simulink model "six_plus_six_AcmsteeringV10_main"  (R2014a)
settings: Solver=FixedStepDiscrete  StartTime=0.0  StopTime=10.0  FixedStep=0.0005  RelTol=1e-3
InitFcn:
  | Veh_Par_wxt
values from neighbouring files (symbols this model uses):
  acc_spdctl = [0 100]    [Veh_Par_wxt.m]
  ag_thr = ecucoder_cal(ag_thr)    [Veh_Par_wxt.m]
  B = 1.8    [Veh_Par_wxt.m]
  bra_em = 100    [Veh_Par_wxt.m]
  bra_pre_gz2 = 100/3    (= 33.3333333333)    [Veh_Par_wxt.m]
  bra_pre_gz34 = 10/3    (= 3.33333333333)    [Veh_Par_wxt.m]
  bra_pre_yd = 10/2    (= 5)    [Veh_Par_wxt.m]
  brakepre_dem_data = [0 1 2 3 4 5 6 7 8 9 10]    [Veh_Par_wxt.m]
  brakeTrq_dem_data = [0 125 251 376 502 627 753 878 1004 1129 1255]    [Veh_Par_wxt.m]
  bratrq_max = 4*1255    (= 5020)    [Veh_Par_wxt.m]
  eff_tran = 0.9    [Veh_Par_wxt.m]
  ESP_switch = ecucoder_cal(ESP_switch)    [Veh_Par_wxt.m]
  G = Mass*g    (= 15696)    [Veh_Par_wxt.m]
  kd1 = ecucoder_cal(kd1)    [Veh_Par_wxt.m]
  kd2 = 0    [Veh_Par_wxt.m]
  ki1 = ecucoder_cal(ki1)    [Veh_Par_wxt.m]
  ki2 = 1    [Veh_Par_wxt.m]
  kp1 = ecucoder_cal(kp1)    [Veh_Par_wxt.m]
  kp2 = 300    [Veh_Par_wxt.m]
  L = L1+L2    (= 2.9)    [Veh_Par_wxt.m]
  premax = 100    [Veh_Par_wxt.m]
  Radius = 0.4572/2    (= 0.2286)    [Veh_Par_wxt.m]
  RC_switch = ecucoder_cal(RC_switch)    [Veh_Par_wxt.m]
  s_opt_yi = 0.15    [Veh_Par_wxt.m]
  s_opt_zhuan = 0.8    [Veh_Par_wxt.m]
  s_opt_zhuan_add = 0.05    [Veh_Par_wxt.m]
  s_opt_zhuan_table = [0.8 0.8 0.3 0.3]    [Veh_Par_wxt.m]
  spd_map_mot = [0 499.85 999.79 1500 2000 2500 3000 3500 4000 4500 4999.8 5999.8]    [Veh_Par_wxt.m]
  spd_spdctl = [0 500]    [Veh_Par_wxt.m]
  speed_thr_park = 5/3.6/Radius*tras_ratio*30/pi    (= 464.143899364)    [Veh_Par_wxt.m]
  TCS_switch = ecucoder_cal(TCS_switch)    [Veh_Par_wxt.m]
  tras_ratio = 8    [Veh_Par_wxt.m]
  trq_map_mot = [70.5 70.012 71.154 65.797 53.917 45.159 38.073 32.685 27.48 17.133 14.949 10.07]    [Veh_Par_wxt.m]
  trqmax_yd = 70.5    [Veh_Par_wxt.m]
  trqmax_zx = 70.5    [Veh_Par_wxt.m]
  trqmaxneg = -70.5    [Veh_Par_wxt.m]
  v_gain = 0.9    [Veh_Par_wxt.m]
  v_table = [0 5 20 100]    [Veh_Par_wxt.m]
  v_thr_park = 5    [Veh_Par_wxt.m]
  zhidong_bianmazhi = [-140000 750000]    [Veh_Par_wxt.m]
  zhidong_down = -140000    [Veh_Par_wxt.m]
  zhidong_up = 750000    [Veh_Par_wxt.m]
  zhidong_youmen = [0 100]    [Veh_Par_wxt.m]
  zhuanxiang_bianmazhi = [-400000 0 400000]    [Veh_Par_wxt.m]
  zhuanxiang_down = -400000    [Veh_Par_wxt.m]
  zhuanxiang_up = 400000    [Veh_Par_wxt.m]
  zhuanxiang_youmen = [-100 0 100]    [Veh_Par_wxt.m]
undefined symbols (not defined in the file or in its folder): ecucoder_acal, guzhang_lf, guzhang_lm, guzhang_lr, guzhang_rf, guzhang_rm, guzhang_rr, myFIS
libraries: simulink x979, ec5744lib x59, fuzblock x2
(part 24 of 27)

== system six_plus_six_AcmsteeringV10_main/MainControl/mode_control/forward/forward/Drive/Subsystem4 ==
  MCU2_3 : Inport
  Bus Selector : BusSelector  OutputSignals=MCU2_3MotorStallingFault,MCU2_3UdcDetectionFault,MCU2_3TempSensorFault,MCU2_3ActiveDischargingFault,MCU2_3ldcSensorFault,MCU2_3luSensorFault,MCU2_3lvSensorFault,MCU2_3FaultLevel,MCU2_3Controllerload,MCU2_3CanCommunicationFault,MCU2_3MemoryFault,MCU2_3DownratingFault,MCU2_3IGBTFault,MCU2_3MotorOverTemp,MCU2_3ControllerOverTemp,MCU2_3MotorOverSpeed,MCU2_3RotaryInverterFault,MCU2_3UnderVoltage,MCU2_3OverVoltage,MCU2_3MotorOverLoad
  Compare To Constant{,1..19} (20 alike) : simulink/Logic and Bit Operations/Compare To Constant  relop===  const=1  OutDataTypeStr=boolean
  Logical Operator : Logic  Operator=OR  Inputs=20  AllPortsSameDT=off  OutDataTypeStr=boolean
  guzhang_rm : Outport
  wires:
  MCU2_3/1 -> Bus Selector/1
  Bus Selector/1 -> Compare To Constant/1  "<MCU2_3MotorStallingFault>"
  Bus Selector/2 -> Compare To Constant1/1  "<MCU2_3UdcDetectionFault>"
  Bus Selector/3 -> Compare To Constant2/1  "<MCU2_3TempSensorFault>"
  Bus Selector/4 -> Compare To Constant3/1  "<MCU2_3ActiveDischargingFault>"
  Bus Selector/5 -> Compare To Constant4/1  "<MCU2_3ldcSensorFault>"
  Bus Selector/6 -> Compare To Constant5/1  "<MCU2_3luSensorFault>"
  Bus Selector/7 -> Compare To Constant6/1  "<MCU2_3lvSensorFault>"
  Bus Selector/8 -> Compare To Constant7/1  "<MCU2_3FaultLevel>"
  Bus Selector/13 -> Compare To Constant12/1  "<MCU2_3IGBTFault>"
  Bus Selector/14 -> Compare To Constant13/1  "<MCU2_3MotorOverTemp>"
  Bus Selector/10 -> Compare To Constant9/1  "<MCU2_3CanCommunicationFault>"
  Bus Selector/16 -> Compare To Constant15/1  "<MCU2_3MotorOverSpeed>"
  Bus Selector/11 -> Compare To Constant10/1  "<MCU2_3MemoryFault>"
  Bus Selector/15 -> Compare To Constant14/1  "<MCU2_3ControllerOverTemp>"
  Bus Selector/12 -> Compare To Constant11/1  "<MCU2_3DownratingFault>"
  Bus Selector/9 -> Compare To Constant8/1  "<MCU2_3Controllerload>"
  Bus Selector/18 -> Compare To Constant17/1  "<MCU2_3UnderVoltage>"
  Bus Selector/20 -> Compare To Constant19/1  "<MCU2_3MotorOverLoad>"
  Bus Selector/19 -> Compare To Constant18/1  "<MCU2_3OverVoltage>"
  Bus Selector/17 -> Compare To Constant16/1  "<MCU2_3RotaryInverterFault>"
  Compare To Constant9/1 -> Logical Operator/10
  Compare To Constant12/1 -> Logical Operator/13
  Compare To Constant11/1 -> Logical Operator/12
  Compare To Constant15/1 -> Logical Operator/16
  Compare To Constant8/1 -> Logical Operator/9
  Compare To Constant10/1 -> Logical Operator/11
  Compare To Constant13/1 -> Logical Operator/14
  Compare To Constant14/1 -> Logical Operator/15
  Compare To Constant1/1 -> Logical Operator/2
  Compare To Constant17/1 -> Logical Operator/18
  Compare To Constant16/1 -> Logical Operator/17
  Compare To Constant18/1 -> Logical Operator/19
  Compare To Constant19/1 -> Logical Operator/20
  Compare To Constant3/1 -> Logical Operator/4
  Compare To Constant2/1 -> Logical Operator/3
  Compare To Constant6/1 -> Logical Operator/7
  Compare To Constant4/1 -> Logical Operator/5
  Compare To Constant5/1 -> Logical Operator/6
  Compare To Constant7/1 -> Logical Operator/8
  Compare To Constant/1 -> Logical Operator/1
  Logical Operator/1 -> guzhang_rm/1

== system six_plus_six_AcmsteeringV10_main/MainControl/mode_control/forward/forward/Drive/Subsystem5 ==
  MCU2_5 : Inport
  Bus Selector : BusSelector  OutputSignals=MCU2_5MotorStallingFault,MCU2_5UdcDetectionFault,MCU2_5TempSensorFault,MCU2_5ActiveDischargingFault,MCU2_5ldcSensorFault,MCU2_5luSensorFault,MCU2_5lvSensorFault,MCU2_5FaultLevel,MCU2_5Controllerload,MCU2_5CanCommunicationFault,MCU2_5MemoryFault,MCU2_5DownratingFault,MCU2_5IGBTFault,MCU2_5MotorOverTemp,MCU2_5ControllerOverTemp,MCU2_5MotorOverSpeed,MCU2_5RotaryInverterFault,MCU2_5UnderVoltage,MCU2_5OverVoltage,MCU2_5MotorOverLoad
  Compare To Constant{,1..19} (20 alike) : simulink/Logic and Bit Operations/Compare To Constant  relop===  const=1  OutDataTypeStr=boolean
  Logical Operator : Logic  Operator=OR  Inputs=20  AllPortsSameDT=off  OutDataTypeStr=boolean
  guzhang_rr : Outport
  wires:
  Logical Operator/1 -> guzhang_rr/1
  Compare To Constant/1 -> Logical Operator/1
  Compare To Constant7/1 -> Logical Operator/8
  Compare To Constant5/1 -> Logical Operator/6
  Compare To Constant4/1 -> Logical Operator/5
  Compare To Constant6/1 -> Logical Operator/7
  Compare To Constant2/1 -> Logical Operator/3
  Compare To Constant3/1 -> Logical Operator/4
  Compare To Constant19/1 -> Logical Operator/20
  Compare To Constant18/1 -> Logical Operator/19
  Compare To Constant16/1 -> Logical Operator/17
  Compare To Constant17/1 -> Logical Operator/18
  Compare To Constant1/1 -> Logical Operator/2
  Compare To Constant14/1 -> Logical Operator/15
  Compare To Constant13/1 -> Logical Operator/14
  Compare To Constant10/1 -> Logical Operator/11
  Compare To Constant8/1 -> Logical Operator/9
  Compare To Constant15/1 -> Logical Operator/16
  Compare To Constant11/1 -> Logical Operator/12
  Compare To Constant12/1 -> Logical Operator/13
  Compare To Constant9/1 -> Logical Operator/10
  Bus Selector/17 -> Compare To Constant16/1  "<MCU2_5RotaryInverterFault>"
  Bus Selector/19 -> Compare To Constant18/1  "<MCU2_5OverVoltage>"
  Bus Selector/20 -> Compare To Constant19/1  "<MCU2_5MotorOverLoad>"
  Bus Selector/18 -> Compare To Constant17/1  "<MCU2_5UnderVoltage>"
  Bus Selector/9 -> Compare To Constant8/1  "<MCU2_5Controllerload>"
  Bus Selector/12 -> Compare To Constant11/1  "<MCU2_5DownratingFault>"
  Bus Selector/15 -> Compare To Constant14/1  "<MCU2_5ControllerOverTemp>"
  Bus Selector/11 -> Compare To Constant10/1  "<MCU2_5MemoryFault>"
  Bus Selector/16 -> Compare To Constant15/1  "<MCU2_5MotorOverSpeed>"
  Bus Selector/10 -> Compare To Constant9/1  "<MCU2_5CanCommunicationFault>"
  Bus Selector/14 -> Compare To Constant13/1  "<MCU2_5MotorOverTemp>"
  Bus Selector/13 -> Compare To Constant12/1  "<MCU2_5IGBTFault>"
  Bus Selector/8 -> Compare To Constant7/1  "<MCU2_5FaultLevel>"
  Bus Selector/7 -> Compare To Constant6/1  "<MCU2_5lvSensorFault>"
  Bus Selector/6 -> Compare To Constant5/1  "<MCU2_5luSensorFault>"
  Bus Selector/5 -> Compare To Constant4/1  "<MCU2_5ldcSensorFault>"
  Bus Selector/4 -> Compare To Constant3/1  "<MCU2_5ActiveDischargingFault>"
  Bus Selector/3 -> Compare To Constant2/1  "<MCU2_5TempSensorFault>"
  Bus Selector/2 -> Compare To Constant1/1  "<MCU2_5UdcDetectionFault>"
  Bus Selector/1 -> Compare To Constant/1  "<MCU2_5MotorStallingFault>"
  MCU2_5/1 -> Bus Selector/1

== matlab function six_plus_six_AcmsteeringV10_main/MainControl/mode_control/forward/forward/Drive/驱动防滑控制TCS/直行TCS/直行/HeartBeat4 ==
  data: life_pre input; life output
function life = fcn(life_pre)
%#codegen
life=single(life_pre+1);
if life>255
    life=single(0);
end
end

== matlab function six_plus_six_AcmsteeringV10_main/MainControl/mode_control/forward/forward/Drive/驱动防滑控制TCS/直行TCS/直行/HeartBeat5 ==
  data: life_pre input; life output
function life = fcn(life_pre)
%#codegen
life=single(life_pre+1);
if life>255
    life=single(0);
end
end

== matlab function six_plus_six_AcmsteeringV10_main/MainControl/mode_control/forward/forward/Brake/HeartBeat4 ==
  data: life_pre input; life output
function life = fcn(life_pre)
%#codegen
life=single(life_pre+1);
if life>255
    life=single(0);
end
end

== matlab function six_plus_six_AcmsteeringV10_main/MainControl/mode_control/neutral/neutral/HeartBeat ==
  data: life_pre input; life output
function life = fcn(life_pre)
%#codegen
life=single(life_pre+1);
if life>255
    life=single(0);
end
end

== matlab function six_plus_six_AcmsteeringV10_main/MainControl/mode_control/backward/backward/Brake/HeartBeat ==
  data: life_pre input; life output
function life = fcn(life_pre)
%#codegen
life=single(life_pre+1);
if life>255
    life=single(0);
end
end

== matlab function six_plus_six_AcmsteeringV10_main/MainControl/mode_control/backward/backward/Brake/Switch Case Action Subsystem/MATLAB Function5 ==
  data: bratrq_dem_lf input; bratrq_dem_lm input; bratrq_dem_lr input; bratrq_dem_rf input; bratrq_dem_rm input; bratrq_dem_rr input; pwr_chg_bat input; bratrq_mot_lf output; bratrq_mot_lm output; pwr_chg_bat1 input; pwr_chg_bat2 input; trqlimL_dig_lf input; bratrq_mot_lr output; bratrq_mot_rf output; bratrq_mot_rm output; bratrq_mot_rr output; trqlimL_dig_lm input; trqlimL_dig_lr input; trqlimL_dig_rf input; trqlimL_dig_rm input; trqlimL_dig_rr input; speed_act_lf input; speed_act_lm input; speed_act_lr input; speed_act_rf input; speed_act_rm input; speed_act_rr input; trqlim_map_lf input; brapre_out_l output; brapre_out_r output; trqlim_map_lm input; trqlim_map_lr input; trqlim_map_rf input; trqlim_map_rm input; trqlim_map_rr input; tras_ratio input; guzhang_lf input; guzhang_lm input; guzhang_lr input; guzhang_rf input; guzhang_rm input; guzhang_rr input
function [bratrq_mot_lf,bratrq_mot_lm,bratrq_mot_lr,bratrq_mot_rf,bratrq_mot_rm,bratrq_mot_rr,brapre_out_l,brapre_out_r] = fcn(bratrq_dem_lf,bratrq_dem_lm,bratrq_dem_lr,bratrq_dem_rf,bratrq_dem_rm,bratrq_dem_rr,pwr_chg_bat,pwr_chg_bat1,pwr_chg_bat2,trqlimL_dig_lf,trqlimL_dig_lm,trqlimL_dig_lr,trqlimL_dig_rf,trqlimL_dig_rm,trqlimL_dig_rr,speed_act_lf,speed_act_lm,speed_act_lr,speed_act_rf,speed_act_rm,speed_act_rr,trqlim_map_lf,trqlim_map_lm,trqlim_map_lr,trqlim_map_rf,trqlim_map_rm,trqlim_map_rr,tras_ratio,guzhang_lf,guzhang_lm,guzhang_lr,guzhang_rf,guzhang_rm,guzhang_rr)
%#codegen pid模块在外面做，里面进行十六种情况的判断，先看一下效果，不能再修改。前轴单独控制，后轴低选控制

bratrq_mot_lf1=single(bratrq_dem_lf/tras_ratio);
bratrq_mot_lf2=single(9549*(pwr_chg_bat/2)/speed_act_lf);
bratrq_mot_lf=single(min(trqlimL_dig_lf,min(bratrq_mot_lf1,bratrq_mot_lf2)));

bratrq_mot_lm1=single(bratrq_dem_lm/tras_ratio);
bratrq_mot_lm2=single(9549*(pwr_chg_bat1/2)/speed_act_lm);
bratrq_mot_lm=single(min(trqlimL_dig_lm,min(bratrq_mot_lm1,bratrq_mot_lm2)));

bratrq_mot_lr1=single(bratrq_dem_lr/tras_ratio);
bratrq_mot_lr2=single(9549*(pwr_chg_bat2/2)/speed_act_lr);
bratrq_mot_lr=single(min(trqlimL_dig_lr,min(bratrq_mot_lr1,bratrq_mot_lr2)));
 
bratrq_mot_rf1=single(bratrq_dem_rf/tras_ratio);
bratrq_mot_rf2=single(9549*(pwr_chg_bat/2)/speed_act_rf);
bratrq_mot_rf=single(min(trqlimL_dig_rf,min(bratrq_mot_rf1,bratrq_mot_rf2)));

bratrq_mot_rm1=single(bratrq_dem_rm/tras_ratio);
bratrq_mot_rm2=single(9549*(pwr_chg_bat1/2)/speed_act_rm);
bratrq_mot_rm=single(min(trqlimL_dig_rm,min(bratrq_mot_rm1,bratrq_mot_rm2)));

bratrq_mot_rr1=single(bratrq_dem_rr/tras_ratio);
bratrq_mot_rr2=single(9549*(pwr_chg_bat2/2)/speed_act_rr);
bratrq_mot_rr=single(min(trqlimL_dig_rr,min(bratrq_mot_rr1,bratrq_mot_rr2)));

brapre_out_l=single(((bratrq_dem_lf+bratrq_dem_lm+bratrq_dem_lr)-(bratrq_mot_lf+bratrq_mot_lm+bratrq_mot_lr)*tras_ratio)/3/150);
brapre_out_r=single(((bratrq_dem_rf+bratrq_dem_rm+bratrq_dem_rr)-(bratrq_mot_rf+bratrq_mot_rm+bratrq_mot_rr)*tras_ratio)/3/150);







bratrq_mot_lf=single(min(bratrq_mot_lf,trqlim_map_lf));%限一下最大值在外特性内，最小值大于0
bratrq_mot_lf=single(max(bratrq_mot_lf,0));
bratrq_mot_lr=single(min(bratrq_mot_lr,trqlim_map_lr));
bratrq_mot_lr=single(max(bratrq_mot_lr,0));
bratrq_mot_rf=single(min(bratrq_mot_rf,trqlim_map_rf));
bratrq_mot_rf=single(max(bratrq_mot_rf,0));
bratrq_mot_rr=single(min(bratrq_mot_rr,trqlim_map_rr));
bratrq_mot_rr=single(max(bratrq_mot_rr,0));

% brapre_out_l=brapre_out_l;
% brapre_out_r=brapre_out_r;
brapre_out_l=single(brapre_out_l*150/125);%第二辆车的制动压力与制动力的关系调整一下。
brapre_out_r=single(brapre_out_r*150/125);

if guzhang_lf==1
    bratrq_mot_lf=single(0);
end
if guzhang_lm==1
    bratrq_mot_lm=single(0);
end
if guzhang_lr==1
    bratrq_mot_lr=single(0);
end
if guzhang_rf==1
    bratrq_mot_rf=single(0);
end
if guzhang_rm==1
    bratrq_mot_rm=single(0);
end
if guzhang_rr==1
    bratrq_mot_rr=single(0);
end

end

== system six_plus_six_AcmsteeringV10_main/MainControl/mode_control/forward/forward/Drive/容错控制 ==
  trq_dem_l : Inport
  trq_dem_r : Inport  Port=2
  trqlim_lf : Inport  Port=3
  trqlim_lm : Inport  Port=4
  trqlim_lr : Inport  Port=5
  trqlim_rf : Inport  Port=6
  trqlim_rm : Inport  Port=7
  trqlim_rr : Inport  Port=8
  guzhang_lf : Inport  Port=9
  guzhang_lm : Inport  Port=10
  guzhang_lr : Inport  Port=11
  guzhang_rf : Inport  Port=12
  guzhang_rm : Inport  Port=13
  guzhang_rr : Inport  Port=14
  Constant : Constant  Value=bra_pre_gz2  OutDataTypeStr=single  SampleTime=-1
  Constant1 : Constant  Value=bra_pre_gz34  OutDataTypeStr=single  SampleTime=-1
  Constant11 : Constant  Value=RC_switch  OutDataTypeStr=single  SampleTime=-1
  Data Type Conversion{,1..5} (6 alike) : DataTypeConversion
  ECCalVar : Constant  InitFcn=ecucoder_acal;  Value=guzhang_lf  OutDataTypeStr=Inherit: Inherit via back propagation  SampleTime=-1
  ECCalVar1 : Constant  InitFcn=ecucoder_acal;  Value=guzhang_lm  OutDataTypeStr=Inherit: Inherit via back propagation  SampleTime=-1
  ECCalVar2 : Constant  InitFcn=ecucoder_acal;  Value=guzhang_lr  OutDataTypeStr=Inherit: Inherit via back propagation  SampleTime=-1
  ECCalVar3 : Constant  InitFcn=ecucoder_acal;  Value=guzhang_rf  OutDataTypeStr=Inherit: Inherit via back propagation  SampleTime=-1
  ECCalVar4 : Constant  InitFcn=ecucoder_acal;  Value=guzhang_rm  OutDataTypeStr=Inherit: Inherit via back propagation  SampleTime=-1
  ECCalVar5 : Constant  InitFcn=ecucoder_acal;  Value=guzhang_rr  OutDataTypeStr=Inherit: Inherit via back propagation  SampleTime=-1
  MATLAB Function : MATLAB Function  TreatAsAtomicUnit=on
  MATLAB Function5 : MATLAB Function  TreatAsAtomicUnit=on
  Terminator : Terminator
  trq_dem_lf : Outport
  trq_dem_lm : Outport  Port=2
  trq_dem_lr : Outport  Port=3
  trq_dem_rf : Outport  Port=4
  trq_dem_rm : Outport  Port=5
  trq_dem_rr : Outport  Port=6
  bra_pre_l : Outport  Port=7
  bra_pre_r : Outport  Port=8
  wires:
  trq_dem_r/1 -> MATLAB Function/2(trq_dem_r)
  trqlim_lr/1 -> MATLAB Function/5(trqlim_lr)
  trq_dem_l/1 -> MATLAB Function/1(trq_dem_l)
  trqlim_rf/1 -> MATLAB Function/6(trqlim_rf)
  trqlim_rr/1 -> MATLAB Function/8(trqlim_rr)
  trqlim_lf/1 -> MATLAB Function/3(trqlim_lf)
  MATLAB Function/1(trq_dem_lf) -> trq_dem_lf/1
  MATLAB Function/3(trq_dem_lr) -> trq_dem_lr/1
  MATLAB Function/4(trq_dem_rf) -> trq_dem_rf/1
  MATLAB Function/6(trq_dem_rr) -> trq_dem_rr/1
  MATLAB Function/7(bra_pre_l) -> bra_pre_l/1
  MATLAB Function/8(bra_pre_r) -> bra_pre_r/1
  Constant/1 -> MATLAB Function/15(bra_pre_gz2)
  Constant1/1 -> MATLAB Function/16(bra_pre_gz34)
  MATLAB Function/9(mode) -> Terminator/1
  trqlim_lm/1 -> MATLAB Function/4(trqlim_lm)
  trqlim_rm/1 -> MATLAB Function/7(trqlim_rm)
  MATLAB Function/2(trq_dem_lm) -> trq_dem_lm/1
  MATLAB Function/5(trq_dem_rm) -> trq_dem_rm/1
  Constant11/1 -> MATLAB Function5/1(RC_switch)
  MATLAB Function5/1(guzhang_lf1) -> Data Type Conversion/1
  MATLAB Function5/2(guzhang_lm1) -> Data Type Conversion1/1
  MATLAB Function5/3(guzhang_lr1) -> Data Type Conversion2/1
  MATLAB Function5/4(guzhang_rf1) -> Data Type Conversion3/1
  MATLAB Function5/6(guzhang_rr1) -> Data Type Conversion5/1
  MATLAB Function5/5(guzhang_rm1) -> Data Type Conversion4/1
  ECCalVar/1 -> MATLAB Function5/2(guzhang_lf)
  ECCalVar1/1 -> MATLAB Function5/3(guzhang_lm)
  ECCalVar2/1 -> MATLAB Function5/4(guzhang_lr)
  ECCalVar3/1 -> MATLAB Function5/5(guzhang_rf)
  ECCalVar4/1 -> MATLAB Function5/6(guzhang_rm)
  ECCalVar5/1 -> MATLAB Function5/7(guzhang_rr)
  Data Type Conversion/1 -> MATLAB Function/9(guzhang_lf)  "guzhang_lf"
  Data Type Conversion1/1 -> MATLAB Function/10(guzhang_lm)  "guzhang_lm"
  Data Type Conversion2/1 -> MATLAB Function/11(guzhang_lr)  "guzhang_lr"
  Data Type Conversion3/1 -> MATLAB Function/12(guzhang_rf)  "guzhang_rf"
  Data Type Conversion4/1 -> MATLAB Function/13(guzhang_rm)  "guzhang_rm"
  Data Type Conversion5/1 -> MATLAB Function/14(guzhang_rr)  "guzhang_rr"

== system six_plus_six_AcmsteeringV10_main/MainControl/mode_control/forward/forward/Drive/左右侧电机分配及功率限制 ==
  Trq_line_dem : Inport
  delta_T_dem : Inport  Port=2
  pwr_dis_bat : Inport  Port=3
  pwr_dis_bat1 : Inport  Port=4
  pwr_dis_bat2 : Inport  Port=5
  speed_act_lf : Inport  Port=6
  speed_act_lm : Inport  Port=7
  speed_act_lr : Inport  Port=8
  speed_act_rf : Inport  Port=9
  speed_act_rm : Inport  Port=10
  speed_act_rr : Inport  Port=11
  TrqLimU_dig_lf : Inport  Port=12
  TrqLimU_dig_lm : Inport  Port=13
  TrqLimU_dig_lr : Inport  Port=14
  TrqLimU_dig_rf : Inport  Port=15
  TrqLimU_dig_rm : Inport  Port=16
  TrqLimU_dig_rr : Inport  Port=17
  Add : Sum
  Add1 : Sum  Inputs=++++++
  Add2 : Sum  Inputs=+++
  Add3 : Sum  Inputs=+++
  Add4 : Sum  Inputs=+++
  Constant : Constant  Value=9549  OutDataTypeStr=single  SampleTime=-1
  Divide : Product  Inputs=**/
  Gain : Gain  Gain=1/6
  Gain1 : Gain  Gain=1/2
  Gain4 : Gain  Gain=1/2
  MATLAB Function : MATLAB Function  TreatAsAtomicUnit=on
  MinMax{,1..8} (9 alike) : MinMax  Inputs=2
  Subtract : Sum  Inputs=+-
  mot_map{,1..5} (6 alike) : Lookup_n-D  NumberOfTableDimensions=1  BreakpointsForDimension1=spd_map_mot  Table=trq_map_mot  InternalRulePriority=Speed  RndMeth=Simplest  InputSameDT=on
  trq_dem_l : Outport
  trq_dem_r : Outport  Port=2
  trqlim_lf : Outport  Port=3
  trqlim_lm : Outport  Port=4
  trqlim_lr : Outport  Port=5
  trqlim_rf : Outport  Port=6
  trqlim_rm : Outport  Port=7
  trqlim_rr : Outport  Port=8
  wires:
  speed_act_rf/1 -> Add1/4, mot_map2/1
  speed_act_lm/1 -> Add1/2, mot_map4/1
  speed_act_rr/1 -> Add1/6, mot_map3/1
  speed_act_lf/1 -> mot_map/1, Add1/1
  Add1/1 -> Gain/1
  Constant/1 -> Divide/1
  Gain/1 -> Divide/3
  Divide/1 -> MinMax/1
  Trq_line_dem/1 -> MinMax/2
  MinMax/1 -> Gain1/1
  Gain1/1 -> Subtract/1, Add/1
  delta_T_dem/1 -> Gain4/1, [delta_T_dem]
  Subtract/1 -> MinMax1/2
  MinMax1/1 -> MATLAB Function/2(trq_dem_l1)
  Add/1 -> MinMax2/2
  MinMax2/1 -> MATLAB Function/4(trq_dem_r1)
  mot_map3/1 -> MinMax3/1
  TrqLimU_dig_rr/1 -> MinMax3/2
  mot_map2/1 -> MinMax4/1
  TrqLimU_dig_rf/1 -> MinMax4/2
  mot_map1/1 -> MinMax5/1
  TrqLimU_dig_lr/1 -> MinMax5/2
  mot_map/1 -> MinMax6/1
  TrqLimU_dig_lf/1 -> MinMax6/2
  MinMax6/1 -> trqlim_lf/1, Add3/1
  MinMax5/1 -> trqlim_lr/1, Add3/3
  MinMax4/1 -> Add2/1, trqlim_rf/1
  MinMax3/1 -> Add2/3, trqlim_rr/1
  Add3/1 -> [trqlim_l]
  [trqlim_l] -> MATLAB Function/1(trqlim_l), MinMax1/1
  Add2/1 -> [trqlim_r]
  [trqlim_r] -> MATLAB Function/3(trqlim_r), MinMax2/1
  [delta_T_dem] -> MATLAB Function/5(delta_T_dem)
  MATLAB Function/1(trq_dem_l) -> trq_dem_l/1
  MATLAB Function/2(trq_dem_r) -> trq_dem_r/1
  Gain4/1 -> Add/2, Subtract/2
  speed_act_lr/1 -> Add1/3, mot_map1/1
  mot_map4/1 -> MinMax7/1
  TrqLimU_dig_lm/1 -> MinMax7/2
  MinMax7/1 -> Add3/2, trqlim_lm/1
  speed_act_rm/1 -> Add1/5, mot_map5/1
  mot_map5/1 -> MinMax8/1
  TrqLimU_dig_rm/1 -> MinMax8/2
  MinMax8/1 -> trqlim_rm/1, Add2/2
  pwr_dis_bat2/1 -> Add4/3
  pwr_dis_bat/1 -> Add4/1
  pwr_dis_bat1/1 -> Add4/2
  Add4/1 -> Divide/2

== system six_plus_six_AcmsteeringV10_main/MainControl/mode_control/forward/forward/Drive/目标直驶力矩确定模块 ==
  acc_dem : Inport
  TrqLimU_dig_lf : Inport  Port=2
  TrqLimU_dig_lm : Inport  Port=3
  TrqLimU_dig_lr : Inport  Port=4
  TrqLimU_dig_rf : Inport  Port=5
  TrqLimU_dig_rm : Inport  Port=6
  TrqLimU_dig_rr : Inport  Port=7
  speed_act_lf : Inport  Port=8
  speed_act_lm : Inport  Port=9
  speed_act_lr : Inport  Port=10
  speed_act_rf : Inport  Port=11
  speed_act_rm : Inport  Port=12
  speed_act_rr : Inport  Port=13
  Add : Sum  Inputs=++++++
  Constant : Constant  Value=3.6  OutDataTypeStr=single  SampleTime=-1
  Constant1 : Constant  Value=Radius  OutDataTypeStr=single  SampleTime=-1
  Constant2 : Constant  Value=30/pi  OutDataTypeStr=single  SampleTime=-1
  Divide : Product  Inputs=*//*
  Gain : Gain  Gain=1/100
  Gain1 : Gain  Gain=tras_ratio
  Ground : Ground
  MinMax{,1..5} (6 alike) : MinMax  Inputs=2
  Product : Product
  Terminator : Terminator
  mot_map{,1..5} (6 alike) : Lookup_n-D  NumberOfTableDimensions=1  BreakpointsForDimension1=spd_map_mot  Table=trq_map_mot  InternalRulePriority=Speed  RndMeth=Simplest  InputSameDT=on
  Trq_line_dem : Outport
  wires:
  Constant1/1 -> Divide/3
  Constant/1 -> Divide/2
  Constant2/1 -> Divide/4
  Divide/1 -> Gain1/1
  TrqLimU_dig_lf/1 -> MinMax/2
  mot_map/1 -> MinMax/1
  TrqLimU_dig_lm/1 -> MinMax1/2
  TrqLimU_dig_rm/1 -> MinMax2/2
  TrqLimU_dig_rr/1 -> MinMax3/2
  Add/1 -> Product/2
  acc_dem/1 -> Gain/1
  Gain/1 -> Product/1
  Ground/1 -> Divide/1
  Gain1/1 -> Terminator/1
  speed_act_lf/1 -> mot_map/1
  speed_act_lm/1 -> mot_map1/1
  speed_act_rm/1 -> mot_map2/1
  speed_act_rr/1 -> mot_map3/1
  mot_map1/1 -> MinMax1/1
  mot_map2/1 -> MinMax2/1
  mot_map3/1 -> MinMax3/1
  Product/1 -> Trq_line_dem/1
  TrqLimU_dig_lr/1 -> MinMax4/2
  mot_map4/1 -> MinMax4/1
  TrqLimU_dig_rf/1 -> MinMax5/2
  speed_act_lr/1 -> mot_map4/1
  speed_act_rf/1 -> mot_map5/1
  mot_map5/1 -> MinMax5/1
  MinMax1/1 -> Add/2
  MinMax/1 -> Add/1
  MinMax4/1 -> Add/3
  MinMax5/1 -> Add/4
  MinMax2/1 -> Add/5
  MinMax3/1 -> Add/6

== system six_plus_six_AcmsteeringV10_main/MainControl/mode_control/forward/forward/Drive/目标转向力矩确定模块 ==
  note: 左转为正，右转为负
  TrqLimU_dig_lf : Inport
  TrqLimU_dig_lm : Inport  Port=2
  TrqLimU_dig_lr : Inport  Port=3
  TrqLimU_dig_rf : Inport  Port=4
  TrqLimU_dig_rm : Inport  Port=5
  TrqLimU_dig_rr : Inport  Port=6
  steer_dem : Inport  Port=7
  umax : Inport  Port=8
  f : Inport  Port=9
  speed_act_lf : Inport  Port=10
  speed_act_lm : Inport  Port=11
  speed_act_lr : Inport  Port=12
  speed_act_rf : Inport  Port=13
  speed_act_rm : Inport  Port=14
  speed_act_rr : Inport  Port=15
  Add : Sum  Inputs=+++
  Add1 : Sum  Inputs=+++
  Add2 : Sum  Inputs=++++++
  Constant : Constant  Value=3.6  OutDataTypeStr=single  SampleTime=-1
  Constant1 : Constant  Value=Radius  OutDataTypeStr=single  SampleTime=-1
  Constant2 : Constant  Value=30/pi  OutDataTypeStr=single  SampleTime=-1
  Constant3 : Constant  Value=G  OutDataTypeStr=single  SampleTime=-1
  Constant4 : Constant  Value=L  OutDataTypeStr=single  SampleTime=-1
  Constant5 : Constant  Value=B  OutDataTypeStr=single  SampleTime=-1
  Constant6 : Constant  Value=eff_tran  OutDataTypeStr=single  SampleTime=-1
  Constant7 : Constant  Value=Radius  OutDataTypeStr=single  SampleTime=-1
  Constant8 : Constant  Value=ag_thr  OutDataTypeStr=single  SampleTime=-1
  Constant9 : Constant  Value=Radius  OutDataTypeStr=single  SampleTime=-1
  Divide : Product  Inputs=*//*
  Gain : Gain  Gain=1/100
  Gain1 : Gain  Gain=tras_ratio
  Gain10 : Gain  Gain=3.6
  Gain2 : Gain  Gain=tras_ratio  OutDataTypeStr=single
  Gain3 : Gain  Gain=1/tras_ratio
  Gain4 : Gain  Gain=tras_ratio  OutDataTypeStr=single
  Gain6 : Gain  Gain=1/6
  Gain7 : Gain  Gain=1/tras_ratio
  Gain8 : Gain  Gain=pi/30
  Gain9 : Gain  Gain=Radius
  Ground : Ground
  MATLAB Function : MATLAB Function  TreatAsAtomicUnit=on
  MATLAB Function1 : MATLAB Function  TreatAsAtomicUnit=on
  MATLAB Function2 : MATLAB Function  TreatAsAtomicUnit=on
  MinMax{,1..3,5..6} (6 alike) : MinMax  Inputs=2
  MinMax4 : MinMax  Function=max  Inputs=2
  Product : Product
  Terminator : Terminator
  mot_map{,1..5} (6 alike) : Lookup_n-D  NumberOfTableDimensions=1  BreakpointsForDimension1=spd_map_mot  Table=trq_map_mot  InternalRulePriority=Speed  RndMeth=Simplest  InputSameDT=on
  delta_Tsteer_dem : Outport
  wires:
  Gain/1 -> Product/1
  Product/1 -> Gain3/1
  [steer_dem] -> Gain/1
  MinMax3/1 -> Add1/2
  MinMax/1 -> Add/1
  MinMax2/1 -> Add1/1
  MinMax1/1 -> Add/2
  TrqLimU_dig_rm/1 -> MinMax3/2
  TrqLimU_dig_rf/1 -> MinMax2/2
  TrqLimU_dig_lm/1 -> MinMax1/2
  mot_map/1 -> MinMax/1
  TrqLimU_dig_lf/1 -> MinMax/2
  Divide/1 -> Gain1/1
  Constant2/1 -> Divide/4
  Constant/1 -> Divide/2
  Constant1/1 -> Divide/3
  steer_dem/1 -> [steer_dem], MATLAB Function/1(steer_dem)
  Constant3/1 -> [G], MATLAB Function/2(G)
  Constant4/1 -> [L], MATLAB Function/3(L)
  Constant5/1 -> [B], MATLAB Function/5(B)
  umax/1 -> [umax], MATLAB Function/4(umax)
  Add/1 -> Gain2/1
  Add1/1 -> Gain4/1
  Constant6/1 -> MATLAB Function/8(eff_tran)
  Constant7/1 -> MATLAB Function/9(Radius)
  f/1 -> MATLAB Function/10(f)
  MATLAB Function/1(Rturn_min) -> MinMax4/1
  [v_act] -> MATLAB Function1/1(v_act)
  Constant8/1 -> MATLAB Function1/2(ag_thr)
  MATLAB Function1/1(Rturn_min_ag) -> MinMax4/2
  [umax] -> MATLAB Function2/1(umax)
  [G] -> MATLAB Function2/2(G)
  [L] -> MATLAB Function2/3(L)
  [B] -> MATLAB Function2/4(B)
  Constant9/1 -> MATLAB Function2/5(Radius)
  MinMax4/1 -> MATLAB Function2/6(Rturn_min_xy)
  MATLAB Function2/1(delta_Tsteer_max) -> Product/2
  Ground/1 -> Divide/1
  Gain2/1 -> MATLAB Function/6(Tpeak_L)
  Gain4/1 -> MATLAB Function/7(Tpeak_R)
  speed_act_lm/1 -> Add2/2, mot_map2/1
  speed_act_rf/1 -> Add2/4, mot_map3/1
  speed_act_rm/1 -> Add2/5, mot_map4/1
  Gain1/1 -> Terminator/1
  speed_act_lf/1 -> Add2/1, mot_map/1
  mot_map2/1 -> MinMax1/1
  mot_map3/1 -> MinMax2/1
  mot_map4/1 -> MinMax3/1
  Gain3/1 -> delta_Tsteer_dem/1
  MinMax5/1 -> Add/3
  TrqLimU_dig_lr/1 -> MinMax5/2
  speed_act_lr/1 -> Add2/3, mot_map1/1
  mot_map1/1 -> MinMax5/1
  MinMax6/1 -> Add1/3
  TrqLimU_dig_rr/1 -> MinMax6/2
  speed_act_rr/1 -> Add2/6, mot_map5/1
  mot_map5/1 -> MinMax6/1
  Add2/1 -> Gain6/1
  Gain6/1 -> Gain7/1
  Gain7/1 -> Gain8/1
  Gain8/1 -> Gain9/1
  Gain9/1 -> Gain10/1
  Gain10/1 -> [v_act]

== system six_plus_six_AcmsteeringV10_main/MainControl/mode_control/forward/forward/Drive/路面状况识别模块 ==
  In1 : Inport
  miu : Inport  Port=2
  slip_ratio : Inport  Port=3
  Signals : Inport  Port=4
  1-D Lookup Table : Lookup_n-D  NumberOfTableDimensions=1  BreakpointsForDimension1=v_table  Table=s_opt_zhuan_table  InternalRulePriority=Speed  RndMeth=Simplest  InputSameDT=on
  Abs{11..14,19..20} (6 alike) : Abs  OutDataTypeStr=single
  Bus Selector8 : BusSelector  OutputSignals=MOTOR.MOTOR1.MCU0.MCU0_SpeedFdk,MOTOR.MOTOR3.MCU0_2.MCU0_2SpeedFdk,MOTOR.MOTOR5.MCU0_4.MCU0_4SpeedFdk,MOTOR.MOTOR2.MCU0_1.MCU0_1SpeedFdk,MOTOR.MOTOR4.MCU0_3.MCU0_3SpeedFdk,MOTOR.MOTOR6.MCU0_5.MCU0_5SpeedFdk
  Constant : Constant  Value=0.9  OutDataTypeStr=single  SampleTime=-1
  Constant1 : Constant  Value=0.05  OutDataTypeStr=single  SampleTime=-1
  Constant2 : Constant  Value=s_opt_zhuan  OutDataTypeStr=single  SampleTime=-1
  Constant3 : Constant  Value=s_opt_yi  OutDataTypeStr=single  SampleTime=-1
  Gain1 : Gain  Gain=1/tras_ratio
  Gain2 : Gain  Gain=pi/30
  Gain3 : Gain  Gain=Radius
  Gain4 : Gain  Gain=3.6
  Gain5 : Gain  Gain=v_gain
  MinMax : MinMax  Inputs=6
  Terminator{,1..3} (4 alike) : Terminator
  路面识别模块 : Subsystem  Commented=on
  umax : Outport
  f : Outport  Port=2
  s_opt_zhuan : Outport  Port=3
  s_opt_yi : Outport  Port=4
  wires:
  Constant/1 -> umax/1
  Constant1/1 -> f/1
  Constant2/1 -> Terminator3/1
  Constant3/1 -> s_opt_yi/1
  In1/1 -> Terminator/1
  miu/1 -> 路面识别模块/1(miu)
  slip_ratio/1 -> 路面识别模块/2(slip_ratio)
  路面识别模块/1(best_slip_ratio) -> Terminator1/1
  路面识别模块/2(max_miu) -> Terminator2/1
  Signals/1 -> Bus Selector8/1
  Abs12/1 -> MinMax/2
  Abs11/1 -> MinMax/1
  Abs13/1 -> MinMax/3
  Abs14/1 -> MinMax/4
  Abs19/1 -> MinMax/5
  Abs20/1 -> MinMax/6
  Bus Selector8/2 -> Abs12/1  "<MCU0_2SpeedFdk>"
  Bus Selector8/1 -> Abs11/1  "<MCU0_SpeedFdk>"
  Bus Selector8/3 -> Abs13/1  "<MCU0_4SpeedFdk>"
  Bus Selector8/4 -> Abs14/1  "<MCU0_1SpeedFdk>"
  Bus Selector8/5 -> Abs19/1  "<MCU0_3SpeedFdk>"
  Bus Selector8/6 -> Abs20/1  "<MCU0_5SpeedFdk>"
  MinMax/1 -> Gain1/1
  Gain1/1 -> Gain2/1
  Gain2/1 -> Gain3/1
  Gain3/1 -> Gain4/1
  Gain4/1 -> Gain5/1
  Gain5/1 -> 1-D Lookup Table/1
  1-D Lookup Table/1 -> s_opt_zhuan/1

== system six_plus_six_AcmsteeringV10_main/MainControl/mode_control/forward/forward/Drive/车辆稳定性控制 ==
  note: 加速度向左为正
  acc_y : Inport
  Action Port : ActionPort  ActionType=case
  Abs : Abs
  Add10 : Sum  Inputs=+-+
  Add2 : Sum  Inputs=+++
  Constant : Constant  Value=ag_thr  OutDataTypeStr=single  SampleTime=-1
  Constant1 : Constant  OutDataTypeStr=int8  SampleTime=-1
  Constant2 : Constant  Value=-1  OutDataTypeStr=int8  SampleTime=-1
  Constant3 : Constant  Value=ESP_switch  OutDataTypeStr=single  SampleTime=-1
  Constant4 : Constant  Value=0  OutDataTypeStr=single  SampleTime=-1
  Gain20 : Gain  Gain=2
  Gain3 : Gain  Gain=1/tras_ratio
  Gain5 : Gain  Gain=kp1  OutDataTypeStr=single
  Gain6 : Gain  Gain=ki1  OutDataTypeStr=single
  Gain7 : Gain  Gain=kd1  OutDataTypeStr=single
  Memory{3..5,13} (4 alike) : Memory  InheritSampleTime=on
  Product : Product  OutDataTypeStr=single
  Subtract1 : Sum  Inputs=+-
  Subtract5 : Sum
  Sum : Sum  Inputs=|+-
  Switch : Switch
  Switch1 : Switch  Criteria=u2 > Threshold  Threshold=0.5
  delta_Twending_dem : Outport
  wires:
  Constant/1 -> Sum/1
  acc_y/1 -> Switch/2, Abs/1  "acc_y"
  Constant1/1 -> Switch/1
  Constant2/1 -> Switch/3
  Switch/1 -> Product/2
  Product/1 -> Gain3/1
  Constant3/1 -> Switch1/2
  Switch1/1 -> delta_Twending_dem/1  "delta_Twending_dem"
  Constant4/1 -> Switch1/3
  Sum/1 -> Memory4/1, Add10/1, Gain6/1, Memory3/1, Subtract1/1
  Gain5/1 -> Add2/1
  Gain6/1 -> Add2/2
  Memory3/1 -> Subtract1/2
  Add10/1 -> Gain7/1
  Gain20/1 -> Add10/2
  Memory5/1 -> Add10/3
  Gain7/1 -> Add2/3
  Subtract1/1 -> Gain5/1
  Memory4/1 -> Memory5/1, Gain20/1
  Add2/1 -> Subtract5/1
  Subtract5/1 -> Product/1, Memory13/1
  Memory13/1 -> Subtract5/2
  Abs/1 -> Sum/2
  Gain3/1 -> Switch1/1

== system six_plus_six_AcmsteeringV10_main/MainControl/mode_control/forward/forward/Drive/车辆稳定性控制1 ==
  Action Port : ActionPort  ActionType=case
  Constant4 : Constant  Value=0  OutDataTypeStr=single  SampleTime=-1
  1 : Outport
  wires:
  Constant4/1 -> 1/1

== system six_plus_six_AcmsteeringV10_main/MainControl/mode_control/forward/forward/Drive/驱动防滑控制TCS ==
  trq_dem_lf : Inport
  trq_dem_lm : Inport  Port=2
  trq_dem_lr : Inport  Port=3
  trq_dem_rf : Inport  Port=4
  trq_dem_rm : Inport  Port=5
  trq_dem_rr : Inport  Port=6
  bra_pre_l : Inport  Port=7
  bra_pre_r : Inport  Port=8
  speed_act_lf : Inport  Port=9
  speed_act_lm : Inport  Port=10
  speed_act_lr : Inport  Port=11
  speed_act_rf : Inport  Port=12
  speed_act_rm : Inport  Port=13
  speed_act_rr : Inport  Port=14
  v_act : Inport  Port=15
  brake_dem : Inport  Port=16
  s_opt_zhuan : Inport  Port=17
  Signals : Inport  Port=18
  直行TCS : Subsystem  TreatAsAtomicUnit=on
  forward_dem : Outport
  wires:
  直行TCS/1(forward_dem) -> forward_dem/1
  trq_dem_lf/1 -> 直行TCS/1(trq_dem_lf)
  trq_dem_lm/1 -> 直行TCS/2(trq_dem_lm)
  trq_dem_lr/1 -> 直行TCS/3(trq_dem_lr)
  trq_dem_rf/1 -> 直行TCS/4(trq_dem_rf)
  trq_dem_rm/1 -> 直行TCS/5(trq_dem_rm)
  trq_dem_rr/1 -> 直行TCS/6(trq_dem_rr)
  bra_pre_l/1 -> 直行TCS/7(bra_pre_l)
  bra_pre_r/1 -> 直行TCS/8(bra_pre_r)
  brake_dem/1 -> 直行TCS/16(brake_dem)
  Signals/1 -> 直行TCS/18(Signals)
  speed_act_rr/1 -> 直行TCS/14(speed_act_rr)
  speed_act_rm/1 -> 直行TCS/13(speed_act_rm)
  v_act/1 -> 直行TCS/15(v_act)
  speed_act_rf/1 -> 直行TCS/12(speed_act_rf)
  speed_act_lr/1 -> 直行TCS/11(speed_act_lr)
  speed_act_lm/1 -> 直行TCS/10(speed_act_lm)
  speed_act_lf/1 -> 直行TCS/9(speed_act_lf)
  s_opt_zhuan/1 -> 直行TCS/17(s_opt_zhuan)

== system six_plus_six_AcmsteeringV10_main/MainControl/mode_control/backward/backward/Drive/路面状况识别模块/路面识别模块 ==
  miu : Inport
  slip_ratio : Inport  Port=2
  Add : Sum  Inputs=+++++
  Add1 : Sum  Inputs=+++++
  Add2 : Sum  Inputs=+++++
  Demux : Demux  Outputs=5
  Display : Display
  Display1 : Display
  Display2 : Display
  Divide : Product  Inputs=*/
  Divide1 : Product  Inputs=/*
  Fuzzy Logic Controller : fuzblock/Fuzzy Logic  Controller  fis=[myFIS]
  Gain : Gain  Gain=0.03
  Gain1 : Gain  Gain=0.05
  Gain2 : Gain  Gain=0.06
  Gain3 : Gain  Gain=0.19
  Gain4 : Gain  Gain=0.14
  Gain5 : Gain  Gain=0.34
  Gain6 : Gain  Gain=0.13
  Gain7 : Gain  Gain=0.80
  Gain8 : Gain  Gain=0.17
  Gain9 : Gain  Gain=1.17
  Mux : Mux  Inputs=2
  Scope : Scope
  Scope1 : Scope
  Scope2 : Scope
      settings: SaveName=ScopeData2
  best_slip_ratio : Outport
  max_miu : Outport  Port=2
  wires:
  Gain6/1 -> Add/4
  Gain4/1 -> Add/3
  Gain/1 -> Add/1
  Demux/1 -> Add1/1, Gain1/1, Gain/1
  Demux/4 -> Add1/4, Gain6/1, Gain7/1
  Add1/1 -> Divide1/1, Divide/2, Display2/1, Scope/1
  Gain5/1 -> Add2/3
  Gain1/1 -> Add2/1
  Gain9/1 -> Add2/5
  Divide/1 -> Display/1, Scope1/1, best_slip_ratio/1
  Gain7/1 -> Add2/4
  Add/1 -> Divide/1
  Gain2/1 -> Add/2
  Gain8/1 -> Add/5
  Demux/2 -> Add1/2, Gain3/1, Gain2/1
  Mux/1 -> Fuzzy Logic Controller/1
  Fuzzy Logic Controller/1 -> Demux/1
  Demux/3 -> Add1/3, Gain5/1, Gain4/1
  Gain3/1 -> Add2/2
  Add2/1 -> Divide1/2
  Divide1/1 -> Display1/1, Scope2/1, max_miu/1
  Demux/5 -> Add1/5, Gain9/1, Gain8/1
  slip_ratio/1 -> Mux/1
  miu/1 -> Mux/2

== system six_plus_six_AcmsteeringV10_main/MainControl/mode_control/backward/backward/Drive/驱动防滑控制TCS/直行TCS ==
  trq_dem_lf : Inport
  trq_dem_lm : Inport  Port=2
  trq_dem_lr : Inport  Port=3
  trq_dem_rf : Inport  Port=4
  trq_dem_rm : Inport  Port=5
  trq_dem_rr : Inport  Port=6
  bra_pre_l : Inport  Port=7
  bra_pre_r : Inport  Port=8
  speed_act_lf : Inport  Port=9
  speed_act_lm : Inport  Port=10
  speed_act_lr : Inport  Port=11
  speed_act_rf : Inport  Port=12
  speed_act_rm : Inport  Port=13
  speed_act_rr : Inport  Port=14
  v_act : Inport  Port=15
  brake_dem : Inport  Port=16
  s_opt_zhuan : Inport  Port=17
  Signals : Inport  Port=18
  Saturation{,1..5} (6 alike) : Saturate  UpperLimit=2  LowerLimit=0  OutDataTypeStr=single
  Subsystem : Subsystem
  Subsystem1 : Subsystem
  Subsystem2 : Subsystem
  Subsystem3 : Subsystem
  Subsystem4 : Subsystem
  Subsystem5 : Subsystem
  Subsystem6 : Subsystem
  Subsystem7 : Subsystem
  直行 : Subsystem  TreatAsAtomicUnit=on
  backward_dem : Outport
  wires:
  直行/1(backward_dem) -> backward_dem/1
  bra_pre_r/1 -> 直行/8(bra_pre_r)
  bra_pre_l/1 -> 直行/7(bra_pre_l)
  trq_dem_rf/1 -> 直行/4(trq_dem_rf)
  trq_dem_lf/1 -> 直行/1(trq_dem_lf)
  trq_dem_lr/1 -> 直行/3(trq_dem_lr)
  trq_dem_lm/1 -> 直行/2(trq_dem_lm)
  trq_dem_rm/1 -> 直行/5(trq_dem_rm)
  trq_dem_rr/1 -> 直行/6(trq_dem_rr)
  brake_dem/1 -> 直行/15(brake_dem)
  Signals/1 -> 直行/17(Signals)
  Subsystem/1(s_act_lf) -> Saturation/1
  speed_act_lf/1 -> Subsystem6/1(speed_act_lf), Subsystem/1(speed_act_lf)
  Saturation/1 -> 直行/9(s_act_lf)
  Subsystem1/1(s_act_lm) -> Saturation1/1
  Saturation1/1 -> 直行/10(s_act_lm)
  speed_act_lm/1 -> Subsystem6/2(speed_act_lm), Subsystem1/1(speed_act_lm)
  Subsystem2/1(s_act_lr) -> Saturation2/1
  Saturation2/1 -> 直行/11(s_act_lr)
  speed_act_lr/1 -> Subsystem6/3(speed_act_lr), Subsystem2/1(speed_act_lr)
  Subsystem3/1(s_act_rf) -> Saturation3/1
  Saturation3/1 -> 直行/12(s_act_rf)
  speed_act_rf/1 -> Subsystem7/1(speed_act_rf), Subsystem3/1(speed_act_rf)
  Subsystem4/1(s_act_rm) -> Saturation4/1
  speed_act_rm/1 -> Subsystem7/2(speed_act_rm), Subsystem4/1(speed_act_rm)
  Saturation4/1 -> 直行/13(s_act_rm)
  Subsystem5/1(s_act_rr) -> Saturation5/1
  Saturation5/1 -> 直行/14(s_act_rr)
  speed_act_rr/1 -> Subsystem7/3(speed_act_rr), Subsystem5/1(speed_act_rr)
  s_opt_zhuan/1 -> 直行/16(s_opt_zhuan)
  Subsystem6/1(v_act_l) -> Subsystem1/2(v_act), Subsystem/2(v_act), Subsystem2/2(v_act)
  Subsystem7/1(v_act_r) -> Subsystem3/2(v_act), Subsystem4/2(v_act), Subsystem5/2(v_act)

== system six_plus_six_AcmsteeringV10_main/MainControl/mode_control/forward/forward/Drive/路面状况识别模块/路面识别模块 ==
  miu : Inport
  slip_ratio : Inport  Port=2
  Add : Sum  Inputs=+++++
  Add1 : Sum  Inputs=+++++
  Add2 : Sum  Inputs=+++++
  Demux : Demux  Outputs=5
  Display : Display
  Display1 : Display
  Display2 : Display
  Divide : Product  Inputs=*/
  Divide1 : Product  Inputs=/*
  Fuzzy Logic Controller : fuzblock/Fuzzy Logic  Controller  fis=[myFIS]
  Gain : Gain  Gain=0.03
  Gain1 : Gain  Gain=0.05
  Gain2 : Gain  Gain=0.06
  Gain3 : Gain  Gain=0.19
  Gain4 : Gain  Gain=0.14
  Gain5 : Gain  Gain=0.34
  Gain6 : Gain  Gain=0.13
  Gain7 : Gain  Gain=0.80
  Gain8 : Gain  Gain=0.17
  Gain9 : Gain  Gain=1.17
  Mux : Mux  Inputs=2
  Scope : Scope
  Scope1 : Scope
  Scope2 : Scope
      settings: SaveName=ScopeData2
  best_slip_ratio : Outport
  max_miu : Outport  Port=2
  wires:
  Gain6/1 -> Add/4
  Gain4/1 -> Add/3
  Gain/1 -> Add/1
  Demux/1 -> Add1/1, Gain1/1, Gain/1
  Demux/4 -> Add1/4, Gain6/1, Gain7/1
  Add1/1 -> Divide1/1, Divide/2, Display2/1, Scope/1
  Gain5/1 -> Add2/3
  Gain1/1 -> Add2/1
  Gain9/1 -> Add2/5
  Divide/1 -> Display/1, Scope1/1, best_slip_ratio/1
  Gain7/1 -> Add2/4
  Add/1 -> Divide/1
  Gain2/1 -> Add/2
  Gain8/1 -> Add/5
  Demux/2 -> Add1/2, Gain3/1, Gain2/1
  Mux/1 -> Fuzzy Logic Controller/1
  Fuzzy Logic Controller/1 -> Demux/1
  Demux/3 -> Add1/3, Gain5/1, Gain4/1
  Gain3/1 -> Add2/2
  Add2/1 -> Divide1/2
  Divide1/1 -> Display1/1, Scope2/1, max_miu/1
  Demux/5 -> Add1/5, Gain9/1, Gain8/1
  slip_ratio/1 -> Mux/1
  miu/1 -> Mux/2

== system six_plus_six_AcmsteeringV10_main/MainControl/mode_control/forward/forward/Drive/驱动防滑控制TCS/直行TCS ==
  trq_dem_lf : Inport
  trq_dem_lm : Inport  Port=2
  trq_dem_lr : Inport  Port=3
  trq_dem_rf : Inport  Port=4
  trq_dem_rm : Inport  Port=5
  trq_dem_rr : Inport  Port=6
  bra_pre_l : Inport  Port=7
  bra_pre_r : Inport  Port=8
  speed_act_lf : Inport  Port=9
  speed_act_lm : Inport  Port=10
  speed_act_lr : Inport  Port=11
  speed_act_rf : Inport  Port=12
  speed_act_rm : Inport  Port=13
  speed_act_rr : Inport  Port=14
  v_act : Inport  Port=15
  brake_dem : Inport  Port=16
  s_opt_zhuan : Inport  Port=17
  Signals : Inport  Port=18
  Saturation{,1..5} (6 alike) : Saturate  UpperLimit=2  LowerLimit=0  OutDataTypeStr=single
  Subsystem : Subsystem
  Subsystem1 : Subsystem
  Subsystem2 : Subsystem
  Subsystem3 : Subsystem
  Subsystem4 : Subsystem
  Subsystem5 : Subsystem
  Subsystem6 : Subsystem
  Subsystem7 : Subsystem
  直行 : Subsystem  TreatAsAtomicUnit=on
  forward_dem : Outport
  wires:
  直行/1(forward_dem) -> forward_dem/1
  bra_pre_r/1 -> 直行/8(bra_pre_r)
  bra_pre_l/1 -> 直行/7(bra_pre_l)
  trq_dem_rf/1 -> 直行/4(trq_dem_rf)
  trq_dem_lf/1 -> 直行/1(trq_dem_lf)
  trq_dem_lr/1 -> 直行/3(trq_dem_lr)
  trq_dem_lm/1 -> 直行/2(trq_dem_lm)
  trq_dem_rm/1 -> 直行/5(trq_dem_rm)
  trq_dem_rr/1 -> 直行/6(trq_dem_rr)
  brake_dem/1 -> 直行/15(brake_dem)
  Signals/1 -> 直行/17(Signals)
  Subsystem/1(s_act_lf) -> Saturation/1  "s_act_lf"
  speed_act_lf/1 -> Subsystem6/1(speed_act_lf), Subsystem/1(speed_act_lf)
  Saturation/1 -> 直行/9(s_act_lf)
  Subsystem1/1(s_act_lm) -> Saturation1/1  "s_act_lm"
  Saturation1/1 -> 直行/10(s_act_lm)
  speed_act_lm/1 -> Subsystem6/2(speed_act_lm), Subsystem1/1(speed_act_lm)
  Subsystem2/1(s_act_lr) -> Saturation2/1  "s_act_lr"
  Saturation2/1 -> 直行/11(s_act_lr)
  speed_act_lr/1 -> Subsystem6/3(speed_act_lr), Subsystem2/1(speed_act_lr)
  Subsystem3/1(s_act_rf) -> Saturation3/1  "s_act_rf"
  Saturation3/1 -> 直行/12(s_act_rf)
  speed_act_rf/1 -> Subsystem7/1(speed_act_rf), Subsystem3/1(speed_act_rf)
  Subsystem4/1(s_act_rm) -> Saturation4/1  "s_act_rm"
  speed_act_rm/1 -> Subsystem7/2(speed_act_rm), Subsystem4/1(speed_act_rm)
  Saturation4/1 -> 直行/13(s_act_rm)
  Subsystem5/1(s_act_rr) -> Saturation5/1  "s_act_rr"
  Saturation5/1 -> 直行/14(s_act_rr)
  speed_act_rr/1 -> Subsystem7/3(speed_act_rr), Subsystem5/1(speed_act_rr)
  s_opt_zhuan/1 -> 直行/16(s_opt_zhuan)
  Subsystem6/1(v_act_l) -> Subsystem/2(v_act), Subsystem1/2(v_act), Subsystem2/2(v_act)
  Subsystem7/1(v_act_r) -> Subsystem5/2(v_act), Subsystem3/2(v_act), Subsystem4/2(v_act)

== system six_plus_six_AcmsteeringV10_main/MainControl/mode_control/backward/backward/Drive/驱动防滑控制TCS/直行TCS/Subsystem ==
  speed_act_lf : Inport
  v_act : Inport  Port=2
  Add : Sum
  Constant : Constant  Value=eps  OutDataTypeStr=single  SampleTime=-1
  Divide : Product  Inputs=*/
  Gain : Gain  Gain=pi/30
  Gain1 : Gain  Gain=Radius
  Gain2 : Gain  Gain=1/3.6
  Gain3 : Gain  Gain=1/tras_ratio
  Subtract : Sum  Inputs=+-
  s_act_lf : Outport
  wires:
  Divide/1 -> s_act_lf/1
  Add/1 -> Divide/2
  Constant/1 -> Add/2
  Subtract/1 -> Divide/1
  Gain1/1 -> Subtract/1, Add/1
  v_act/1 -> Gain2/1
  Gain/1 -> Gain1/1
  speed_act_lf/1 -> Gain3/1
  Gain3/1 -> Gain/1
  Gain2/1 -> Subtract/2

== system six_plus_six_AcmsteeringV10_main/MainControl/mode_control/backward/backward/Drive/驱动防滑控制TCS/直行TCS/Subsystem1 ==
  speed_act_lm : Inport
  v_act : Inport  Port=2
  Add : Sum
  Constant : Constant  Value=eps  OutDataTypeStr=single  SampleTime=-1
  Divide : Product  Inputs=*/
  Gain : Gain  Gain=pi/30
  Gain1 : Gain  Gain=Radius
  Gain2 : Gain  Gain=1/3.6
  Gain3 : Gain  Gain=1/tras_ratio
  Subtract : Sum  Inputs=+-
  s_act_lm : Outport
  wires:
  Gain2/1 -> Subtract/2
  Gain3/1 -> Gain/1
  speed_act_lm/1 -> Gain3/1
  Gain/1 -> Gain1/1
  v_act/1 -> Gain2/1
  Gain1/1 -> Add/1, Subtract/1
  Subtract/1 -> Divide/1
  Constant/1 -> Add/2
  Add/1 -> Divide/2
  Divide/1 -> s_act_lm/1

== system six_plus_six_AcmsteeringV10_main/MainControl/mode_control/backward/backward/Drive/驱动防滑控制TCS/直行TCS/Subsystem2 ==
  speed_act_lr : Inport
  v_act : Inport  Port=2
  Add : Sum
  Constant : Constant  Value=eps  OutDataTypeStr=single  SampleTime=-1
  Divide : Product  Inputs=*/
  Gain : Gain  Gain=pi/30
  Gain1 : Gain  Gain=Radius
  Gain2 : Gain  Gain=1/3.6
  Gain3 : Gain  Gain=1/tras_ratio
  Subtract : Sum  Inputs=+-
  s_act_lr : Outport
  wires:
  Gain2/1 -> Subtract/2
  Gain3/1 -> Gain/1
  speed_act_lr/1 -> Gain3/1
  Gain/1 -> Gain1/1
  v_act/1 -> Gain2/1
  Gain1/1 -> Add/1, Subtract/1
  Subtract/1 -> Divide/1
  Constant/1 -> Add/2
  Add/1 -> Divide/2
  Divide/1 -> s_act_lr/1

== system six_plus_six_AcmsteeringV10_main/MainControl/mode_control/backward/backward/Drive/驱动防滑控制TCS/直行TCS/Subsystem3 ==
  speed_act_rf : Inport
  v_act : Inport  Port=2
  Add : Sum
  Constant : Constant  Value=eps  OutDataTypeStr=single  SampleTime=-1
  Divide : Product  Inputs=*/
  Gain : Gain  Gain=pi/30
  Gain1 : Gain  Gain=Radius
  Gain2 : Gain  Gain=1/3.6
  Gain3 : Gain  Gain=1/tras_ratio
  Subtract : Sum  Inputs=+-
  s_act_rf : Outport
  wires:
  Divide/1 -> s_act_rf/1
  Add/1 -> Divide/2
  Constant/1 -> Add/2
  Subtract/1 -> Divide/1
  Gain1/1 -> Subtract/1, Add/1
  v_act/1 -> Gain2/1
  Gain/1 -> Gain1/1
  speed_act_rf/1 -> Gain3/1
  Gain3/1 -> Gain/1
  Gain2/1 -> Subtract/2

== system six_plus_six_AcmsteeringV10_main/MainControl/mode_control/backward/backward/Drive/驱动防滑控制TCS/直行TCS/Subsystem4 ==
  speed_act_rm : Inport
  v_act : Inport  Port=2
  Add : Sum
  Constant : Constant  Value=eps  OutDataTypeStr=single  SampleTime=-1
  Divide : Product  Inputs=*/
  Gain : Gain  Gain=pi/30
  Gain1 : Gain  Gain=Radius
  Gain2 : Gain  Gain=1/3.6
  Gain3 : Gain  Gain=1/tras_ratio
  Subtract : Sum  Inputs=+-
  s_act_rm : Outport
  wires:
  Gain2/1 -> Subtract/2
  Gain3/1 -> Gain/1
  speed_act_rm/1 -> Gain3/1
  Gain/1 -> Gain1/1
  v_act/1 -> Gain2/1
  Gain1/1 -> Add/1, Subtract/1
  Subtract/1 -> Divide/1
  Constant/1 -> Add/2
  Add/1 -> Divide/2
  Divide/1 -> s_act_rm/1

== system six_plus_six_AcmsteeringV10_main/MainControl/mode_control/backward/backward/Drive/驱动防滑控制TCS/直行TCS/Subsystem5 ==
  speed_act_rr : Inport
  v_act : Inport  Port=2
  Add : Sum
  Constant : Constant  Value=eps  OutDataTypeStr=single  SampleTime=-1
  Divide : Product  Inputs=*/
  Gain : Gain  Gain=pi/30
  Gain1 : Gain  Gain=Radius
  Gain2 : Gain  Gain=1/3.6
  Gain3 : Gain  Gain=1/tras_ratio
  Subtract : Sum  Inputs=+-
  s_act_rr : Outport
  wires:
  Divide/1 -> s_act_rr/1
  Add/1 -> Divide/2
  Constant/1 -> Add/2
  Subtract/1 -> Divide/1
  Gain1/1 -> Subtract/1, Add/1
  v_act/1 -> Gain2/1
  Gain/1 -> Gain1/1
  speed_act_rr/1 -> Gain3/1
  Gain3/1 -> Gain/1
  Gain2/1 -> Subtract/2

== system six_plus_six_AcmsteeringV10_main/MainControl/mode_control/backward/backward/Drive/驱动防滑控制TCS/直行TCS/Subsystem6 ==
  speed_act_lf : Inport
  speed_act_lm : Inport  Port=2
  speed_act_lr : Inport  Port=3
  Gain : Gain  Gain=1/tras_ratio
  Gain1 : Gain  Gain=pi/30
  Gain2 : Gain  Gain=Radius
  Gain3 : Gain  Gain=3.6
  Gain4 : Gain  Gain=v_gain
  MinMax : MinMax  Inputs=3
  v_act_l : Outport
  wires:
  speed_act_lm/1 -> MinMax/2
  speed_act_lr/1 -> MinMax/3
  speed_act_lf/1 -> MinMax/1
  MinMax/1 -> Gain/1
  Gain/1 -> Gain1/1
  Gain1/1 -> Gain2/1
  Gain2/1 -> Gain3/1
  Gain3/1 -> Gain4/1
  Gain4/1 -> v_act_l/1

== system six_plus_six_AcmsteeringV10_main/MainControl/mode_control/backward/backward/Drive/驱动防滑控制TCS/直行TCS/Subsystem7 ==
  speed_act_rf : Inport
  speed_act_rm : Inport  Port=2
  speed_act_rr : Inport  Port=3
  Gain : Gain  Gain=1/tras_ratio
  Gain1 : Gain  Gain=pi/30
  Gain2 : Gain  Gain=Radius
  Gain3 : Gain  Gain=3.6
  Gain4 : Gain  Gain=v_gain
  MinMax : MinMax  Inputs=3
  v_act_r : Outport
  wires:
  Gain4/1 -> v_act_r/1
  Gain3/1 -> Gain4/1
  Gain2/1 -> Gain3/1
  Gain1/1 -> Gain2/1
  Gain/1 -> Gain1/1
  MinMax/1 -> Gain/1
  speed_act_rf/1 -> MinMax/1
  speed_act_rr/1 -> MinMax/3
  speed_act_rm/1 -> MinMax/2
